simulink model "soc"  (R2025b)
settings: Solver=FixedStepDiscrete  StartTime=0.0  StopTime=10  FixedStep=0.01  RelTol=1e-3
PreLoadFcn:
  | % === Get the current model's directory ===
  | modelFullPath = get_param(bdroot, 'FileName');
  | modelDir = fileparts(modelFullPath);
  | 
  | 
  | % === Get the project root folder ===
  | projectRoot = fileparts(modelDir);
  | 
  | 
  | % === Add key folders to path ===
  | addpath(fullfile(projectRoot, 'ReferenceSubsystems'));
  | %addpath(fullfile(projectRoot, 'Docs'));
  | addpath(fullfile(projectRoot, 'design'));
  | 
  | 
  | % Load lookup table script
  | %run('Lookuptable.m');
  | 
  | 
  | 
  | 
PostLoadFcn:
  | float32 = Simulink.AliasType;
  | 
  | float32.BaseType = 'single';
  | 
  | float32.HeaderFile = 'Platform_Types.h';
  | 
  | assignin('base', 'float32', float32);
values from neighbouring files (symbols this model uses):
  Battsm_State_t : value not decoded    [soc.sldd]
  FRACTION_TO_PERCENT = 100.0    [soc.sldd]
  KeSoc_A_RestingCurrent = 4.0    [soc.sldd]
  KeSoc_frc_BotmOfDchRst = 0.0    [soc.sldd]
  KeSoc_frc_LowSocResetThd = 0.12    [soc.sldd]
  KeSoc_frc_LowSocSetThd = 0.1    [soc.sldd]
  KeSoc_frc_SocMaxLim = 1.0    [soc.sldd]
  KeSoc_frc_SocMinLim = 0.0    [soc.sldd]
  KeSoc_frc_TopOfChrgRst = 1.0    [soc.sldd]
  KeSoc_frc_UserSocMaxLim = 0.99    [soc.sldd]
  KeSoc_frc_UserSocMinLim = 0.014    [soc.sldd]
  KeSoc_nu_EpsVal = 2.2204460492503131E-16    [soc.sldd]
  KeSoc_nu_RestTauFactor = 3.0    [soc.sldd]
  KeSoc_sec_SampleTime = 0.01    [soc.sldd]
  KeSoc_sec_SocBodSetTime = 0.0    [soc.sldd]
  KeSoc_sec_SocTocSetTime = 0.0    [soc.sldd]
  KeSoc_V_BodMinCellVolt = 2.993    [soc.sldd]
  KeSoc_V_TocAvrgCellVolt = 4.5    [soc.sldd]
  KeSoc_V_TocMaxCellVolt = 4.5    [soc.sldd]
  PERCENT_TO_FRACTION = 0.01    [soc.sldd]
  SEC_TO_MILLISEC = 1000.0    [soc.sldd]
  SOC_NUM_OF_CELLS = 8.0    [soc.sldd]
  Soc_State_t : value not decoded    [soc.sldd]
libraries: simulink x25
(part 2 of 2)

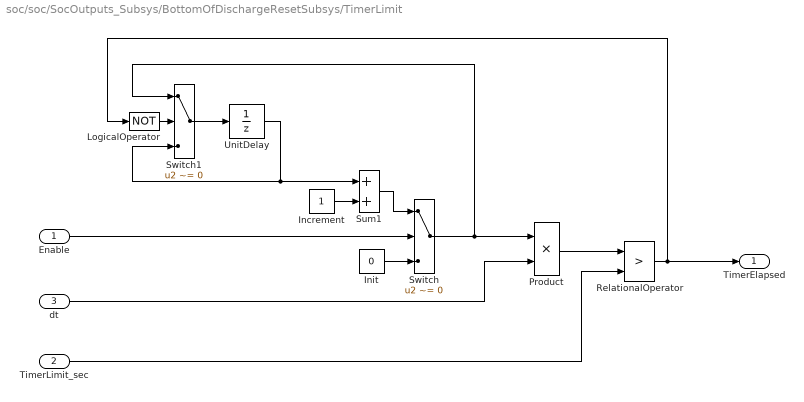
== system soc/soc/SocOutputs_Subsys/BottomOfDischargeResetSubsys/TimerLimit ==
  Enable : Inport  OutDataTypeStr=boolean
  TimerLimit_sec : Inport  Port=2
  dt : Inport  Port=3
  Increment : Constant  OutDataTypeStr=single  SampleTime=-1  FramePeriod=-1
  Init : Constant  Value=0  OutDataTypeStr=single  SampleTime=-1  FramePeriod=-1
  LogicalOperator : Logic  Operator=NOT  AllPortsSameDT=off  OutDataTypeStr=boolean
  Product : Product
  RelationalOperator : RelationalOperator  Tag=struct('comment',struct('text','','placement',1),'logdata',struct('maxnumvals',inf,'plotchannels',[],'stepsize',0,'downsampling',1,'loggingmode',3,'channels',1),'operator','>','output',struct('class','default','type','Bool','description','','address','','unit','','name','$S_$B'),'date',731828.013278403)  Operator=>  OutDataTypeStr=boolean
  Sum1 : Sum  Tag=struct('comment',struct('text','','placement',1),'logdata',struct('maxnumvals',inf,'plotchannels',[],'stepsize',0,'downsampling',1,'loggingmode',3,'channels',1),'output',struct('width',1,'name','$S_$B','unit','','type','Int16','offset',0,'max',NaN,'min',NaN,'freeze',1,'lsb',0.01,'arb',1,'class','default','address','','description','','autoscalingmode',1,'lowerheadroom',1,'upperheadroom',1,'headroomunit','bit','checkmin',0,'checkmax',1,'show',0),'inputs','++','date',731828.013278981)  InputSameDT=on  OutDataTypeStr=Inherit: Same as first input
  Switch : Switch  Tag=struct('comment',struct('text','','placement',1),'logdata',struct('maxnumvals',inf,'plotchannels',[],'stepsize',0,'downsampling',1,'loggingmode',3,'channels',1),'output',struct('width',1,'name','$S_$B','unit','','type','Int16','offset',0,'max',NaN,'min',NaN,'freeze',1,'lsb',0.01,'arb',1,'class','default','address','','description','','autoscalingmode',1,'lowerheadroom',1,'upperheadroom',1,'headroomunit','bit','checkmin',0,'checkmax',0,'show',0),'threshold',struct('width',1,'name','$S_$B_threshold','unit','','type','Int16','offset',0,'max',NaN,'min',NaN,'freeze',1,'lsb',1,'arb',0,'class','default','address','','description','','value','1','scalar',0),'date',731832.69671603)  Criteria=u2 ~= 0  OutDataTypeStr=Inherit: Inherit via back propagation  SaturateOnIntegerOverflow=off
      settings: AttributesFormatString=<Threshold = %<Threshold>>
  Switch1 : Switch  Tag=struct('comment',struct('text','','placement',1),'logdata',struct('maxnumvals',inf,'plotchannels',[],'stepsize',0,'downsampling',1,'loggingmode',3,'channels',1),'output',struct('width',1,'name','$S_$B','unit','','type','Int16','offset',0,'max',NaN,'min',NaN,'freeze',1,'lsb',0.01,'arb',1,'class','default','address','','description','','autoscalingmode',1,'lowerheadroom',1,'upperheadroom',1,'headroomunit','bit','checkmin',0,'checkmax',0,'show',0),'threshold',struct('width',1,'name','$S_$B_threshold','unit','','type','Int16','offset',0,'max',NaN,'min',NaN,'freeze',1,'lsb',1,'arb',0,'class','default','address','','description','','value','1','scalar',0),'date',731832.69671603)  Criteria=u2 ~= 0  OutDataTypeStr=Inherit: Inherit via back propagation  SaturateOnIntegerOverflow=off
      settings: AttributesFormatString=<Threshold = %<Threshold>>
  UnitDelay : UnitDelay  SampleTime=-1  HasFrameUpgradeWarning=on
      settings: AttributesFormatString=<IC: %<InitialCondition>>
  TimerElapsed : Outport  OutDataTypeStr=boolean  VectorParamsAs1DForOutWhenUnconnected=off
      settings: AttributesFormatString=|
      | <IC: %<InitialOutput>>
      | <%<OutputWhenDisabled>>
  wires:
  Increment/1 -> Sum1/2
  TimerLimit_sec/1 -> RelationalOperator/2
  RelationalOperator/1 -> LogicalOperator/1, TimerElapsed/1
  Switch1/1 -> UnitDelay/1
  dt/1 -> Product/2
  Init/1 -> Switch/3
  UnitDelay/1 -> Sum1/1, Switch1/3
  Sum1/1 -> Switch/1
  Product/1 -> RelationalOperator/1
  LogicalOperator/1 -> Switch1/2
  Switch/1 -> Product/1, Switch1/1
  Enable/1 -> Switch/2

== system soc/soc/SocOutputs_Subsys/CalculatePackSoc_Subsys/CapacityRemaining ==
  VaSoc_pct_CellSoc : Inport
  VaSoc_frc_CellSohc : Inport  Port=2
  Constant : Constant  Value=KeSoc_frc_SocMinLim
  Min1 : MinMax  OutMin=0.01  OutMax=1
  Product : Product
  Subtract : Sum  Inputs=+-
  LeSoc_nu_CapcRemaining : Outport  OutMin=0.01  OutMax=1
  wires:
  VaSoc_pct_CellSoc/1 -> Subtract/1
  Constant/1 -> Subtract/2
  Subtract/1 -> Product/1
  VaSoc_frc_CellSohc/1 -> Product/2
  Product/1 -> Min1/1
  Min1/1 -> LeSoc_nu_CapcRemaining/1  "LeSoc_nu_CapcRemaining"

== system soc/soc/SocOutputs_Subsys/CalculatePackSoc_Subsys/CapacityToFullCharge ==
  VaSoc_pct_CellSoc : Inport
  VaSoc_frc_CellSohc : Inport  Port=2
  KeSoc_frc_SocMaxLim : Constant  Value=KeSoc_frc_SocMaxLim
  Min : MinMax  OutMin=0.01  OutMax=1
  Product : Product
  Subtract : Sum  Inputs=+-
  LeSoc_frc_CapcToFullChrg : Outport  OutMin=0.01  OutMax=1
  wires:
  KeSoc_frc_SocMaxLim/1 -> Subtract/1
  VaSoc_pct_CellSoc/1 -> Subtract/2
  Subtract/1 -> Product/1
  VaSoc_frc_CellSohc/1 -> Product/2
  Product/1 -> Min/1
  Min/1 -> LeSoc_frc_CapcToFullChrg/1  "LeSoc_frc_CapcToFullChrg"

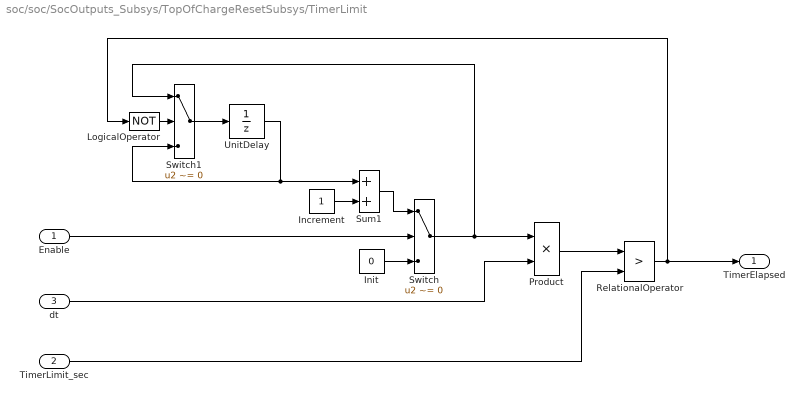
== system soc/soc/SocOutputs_Subsys/TopOfChargeResetSubsys/TimerLimit ==
  Enable : Inport  OutDataTypeStr=boolean
  TimerLimit_sec : Inport  Port=2
  dt : Inport  Port=3
  Increment : Constant  OutDataTypeStr=single  SampleTime=-1  FramePeriod=-1
  Init : Constant  Value=0  OutDataTypeStr=single  SampleTime=-1  FramePeriod=-1
  LogicalOperator : Logic  Operator=NOT  AllPortsSameDT=off  OutDataTypeStr=boolean
  Product : Product
  RelationalOperator : RelationalOperator  Tag=struct('comment',struct('text','','placement',1),'logdata',struct('maxnumvals',inf,'plotchannels',[],'stepsize',0,'downsampling',1,'loggingmode',3,'channels',1),'operator','>','output',struct('class','default','type','Bool','description','','address','','unit','','name','$S_$B'),'date',731828.013278403)  Operator=>  OutDataTypeStr=boolean
  Sum1 : Sum  Tag=struct('comment',struct('text','','placement',1),'logdata',struct('maxnumvals',inf,'plotchannels',[],'stepsize',0,'downsampling',1,'loggingmode',3,'channels',1),'output',struct('width',1,'name','$S_$B','unit','','type','Int16','offset',0,'max',NaN,'min',NaN,'freeze',1,'lsb',0.01,'arb',1,'class','default','address','','description','','autoscalingmode',1,'lowerheadroom',1,'upperheadroom',1,'headroomunit','bit','checkmin',0,'checkmax',1,'show',0),'inputs','++','date',731828.013278981)  InputSameDT=on  OutDataTypeStr=Inherit: Same as first input
  Switch : Switch  Tag=struct('comment',struct('text','','placement',1),'logdata',struct('maxnumvals',inf,'plotchannels',[],'stepsize',0,'downsampling',1,'loggingmode',3,'channels',1),'output',struct('width',1,'name','$S_$B','unit','','type','Int16','offset',0,'max',NaN,'min',NaN,'freeze',1,'lsb',0.01,'arb',1,'class','default','address','','description','','autoscalingmode',1,'lowerheadroom',1,'upperheadroom',1,'headroomunit','bit','checkmin',0,'checkmax',0,'show',0),'threshold',struct('width',1,'name','$S_$B_threshold','unit','','type','Int16','offset',0,'max',NaN,'min',NaN,'freeze',1,'lsb',1,'arb',0,'class','default','address','','description','','value','1','scalar',0),'date',731832.69671603)  Criteria=u2 ~= 0  OutDataTypeStr=Inherit: Inherit via back propagation  SaturateOnIntegerOverflow=off
      settings: AttributesFormatString=<Threshold = %<Threshold>>
  Switch1 : Switch  Tag=struct('comment',struct('text','','placement',1),'logdata',struct('maxnumvals',inf,'plotchannels',[],'stepsize',0,'downsampling',1,'loggingmode',3,'channels',1),'output',struct('width',1,'name','$S_$B','unit','','type','Int16','offset',0,'max',NaN,'min',NaN,'freeze',1,'lsb',0.01,'arb',1,'class','default','address','','description','','autoscalingmode',1,'lowerheadroom',1,'upperheadroom',1,'headroomunit','bit','checkmin',0,'checkmax',0,'show',0),'threshold',struct('width',1,'name','$S_$B_threshold','unit','','type','Int16','offset',0,'max',NaN,'min',NaN,'freeze',1,'lsb',1,'arb',0,'class','default','address','','description','','value','1','scalar',0),'date',731832.69671603)  Criteria=u2 ~= 0  OutDataTypeStr=Inherit: Inherit via back propagation  SaturateOnIntegerOverflow=off
      settings: AttributesFormatString=<Threshold = %<Threshold>>
  UnitDelay : UnitDelay  SampleTime=-1  HasFrameUpgradeWarning=on
      settings: AttributesFormatString=<IC: %<InitialCondition>>
  TimerElapsed : Outport  OutDataTypeStr=boolean  VectorParamsAs1DForOutWhenUnconnected=off
      settings: AttributesFormatString=|
      | <IC: %<InitialOutput>>
      | <%<OutputWhenDisabled>>
  wires:
  Increment/1 -> Sum1/2
  TimerLimit_sec/1 -> RelationalOperator/2
  RelationalOperator/1 -> LogicalOperator/1, TimerElapsed/1
  Switch1/1 -> UnitDelay/1
  dt/1 -> Product/2
  Init/1 -> Switch/3
  UnitDelay/1 -> Sum1/1, Switch1/3
  Sum1/1 -> Switch/1
  Product/1 -> RelationalOperator/1
  LogicalOperator/1 -> Switch1/2
  Switch/1 -> Product/1, Switch1/1
  Enable/1 -> Switch/2

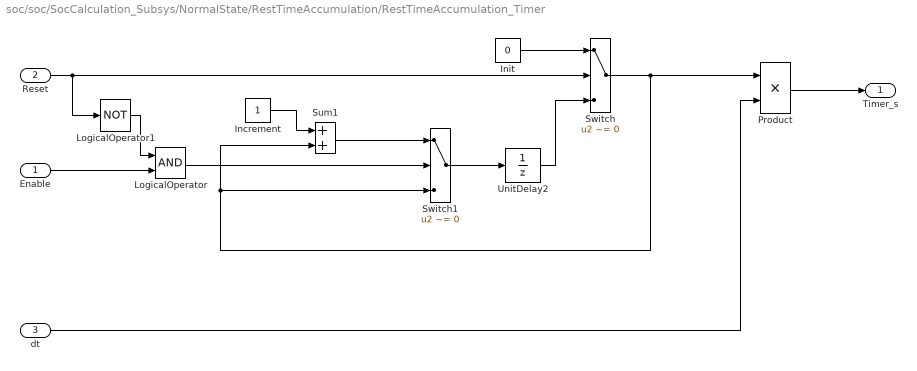
== system soc/soc/SocCalculation_Subsys/NormalState/RestTimeAccumulation/RestTimeAccumulation_Timer ==
  Enable : Inport
  Reset : Inport  Port=2
  dt : Inport  Port=3
  Increment : Constant  OutDataTypeStr=single  SampleTime=-1  FramePeriod=-1
  Init : Constant  Value=0  OutDataTypeStr=single  SampleTime=-1  FramePeriod=-1
  LogicalOperator : Logic  AllPortsSameDT=off  OutDataTypeStr=boolean
  LogicalOperator1 : Logic  Operator=NOT  AllPortsSameDT=off  OutDataTypeStr=boolean
  Product : Product
  Sum1 : Sum  Tag=struct('comment',struct('text','','placement',1),'logdata',struct('maxnumvals',inf,'plotchannels',[],'stepsize',0,'downsampling',1,'loggingmode',3,'channels',1),'output',struct('width',1,'name','$S_$B','unit','','type','Int16','offset',0,'max',NaN,'min',NaN,'freeze',1,'lsb',0.01,'arb',1,'class','default','address','','description','','autoscalingmode',1,'lowerheadroom',1,'upperheadroom',1,'headroomunit','bit','checkmin',0,'checkmax',1,'show',0),'inputs','++','date',731828.013278981)  InputSameDT=on  OutDataTypeStr=Inherit: Same as first input
  Switch : Switch  Criteria=u2 ~= 0  OutDataTypeStr=Inherit: Inherit via back propagation  SaturateOnIntegerOverflow=off
      settings: AttributesFormatString=<Threshold = %<Threshold>>
  Switch1 : Switch  Criteria=u2 ~= 0  OutDataTypeStr=Inherit: Inherit via back propagation  SaturateOnIntegerOverflow=off
      settings: AttributesFormatString=<Threshold = %<Threshold>>
  UnitDelay2 : UnitDelay  SampleTime=-1  HasFrameUpgradeWarning=on
      settings: AttributesFormatString=<IC: %<InitialCondition>>
  Timer_s : Outport  OutDataTypeStr=single  InitialOutput=[0]  VectorParamsAs1DForOutWhenUnconnected=off
      settings: AttributesFormatString=|
      | <IC: %<InitialOutput>>
      | <%<OutputWhenDisabled>>
  wires:
  Enable/1 -> LogicalOperator/2
  Reset/1 -> Switch/2, LogicalOperator1/1
  dt/1 -> Product/2
  Increment/1 -> Sum1/1
  Switch/1 -> Product/1, Sum1/2, Switch1/3
  Switch1/1 -> UnitDelay2/1
  LogicalOperator1/1 -> LogicalOperator/1
  Sum1/1 -> Switch1/1
  Product/1 -> Timer_s/1
  LogicalOperator/1 -> Switch1/2
  Init/1 -> Switch/1
  UnitDelay2/1 -> Switch/3

== stateflow chart soc/SocStateMachine_Subsys/SOC_StateMachine_Chart ==
  note: SOC State Machine:
  state INIT_STATE
    en:
    LeSoc_nu_SocSt=Soc_State_t.SOC_STATE_INIT;
    LeSoc_bi_SocInNormalStateFlg=false;
  note: SOC state machine description:
      |
      | SOC States: SOC_STATE_INIT -0 (Default state)
      | SOC_STATE_RESET - 1
      | SOC_STATE_CORRECTION_ON_WAKE - 2
      | SOC_STATE_NORMAL - 3
      |
      | INIT STATE:
      | This is the default state where the algorithm initializes the SOC values using the data imported from NVM.
      | Based on the NeSoc_bi_NvmImprtScsf flag and the current battery state, the state machine transitions to either SOC_Correction_on_Wake or SOC_Reset.
      |
      | SOC RESET STATE:
      | If the NVM import fails, the SOC values are reset or reinitialized using OCV-based estimates, and the rest time is set to zero.
      | The system then transitions to the Normal state once the battery enters Charge or Drive mode.
      |
      | SOC CORRECTION ON WAKE STATE:
      | If the NVM import is successful, the algorithm checks for any previously accumulated rest time that may require SOC correction before entering the Normal state.
      | If the rest time is sufficiently long, SOC correction is performed; otherwise, the SOC value imported from NVM is retained as the initial SOC.
      | The state transitions to Normal when the battery is in Charge or Drive mode.
      |
      | NORMAL STATE:
      | In this state, SOC is computed using the coulomb counting method.
      | If the battery enters a rest condition, the rest time is accumulated.
      | Once the accumulated rest time exceeds the defined threshold, SOC correction is performed, and the updated value is stored
  state CORRECTION_ON_WAKE_STATE
    en:
    LeSoc_nu_SocSt=Soc_State_t.SOC_STATE_CORRECTION_ON_WAKE;
  state RESET_STATE
    en:
    LeSoc_nu_SocSt=Soc_State_t.SOC_STATE_RESET;
  state NORMAL_STATE
    en:
    LeSoc_nu_SocSt=Soc_State_t.SOC_STATE_NORMAL;
    du:
    LeSoc_bi_SocInNormalStateFlg=true;
    if LeSoc_bi_RestCorrCmpFlg
    LeSoc_bi_CcRst = true;
    else
    LeSoc_bi_CcRst = false;
    end
  (default) -> INIT_STATE
  INIT_STATE -> (junction 8) [order 1] : [NeSoc_bi_NvmImprtScsf == true &&...
      | [ VeBattsm_nu_BattState == Battsm_State_t.BATTSM_STATE_STANDBY_INIT ||...
      | VeBattsm_nu_BattState == Battsm_State_t.BATTSM_STATE_STANDBY_NOT_READY ||...
      | VeBattsm_nu_BattState == Battsm_State_t.BATTSM_STATE_STANDBY_READY]]
  (junction 8) -> CORRECTION_ON_WAKE_STATE
  INIT_STATE -> RESET_STATE [order 2] : [NeSoc_bi_NvmImprtScsf ~= true &&...
      | [ VeBattsm_nu_BattState == Battsm_State_t.BATTSM_STATE_STANDBY_INIT ||...
      | VeBattsm_nu_BattState == Battsm_State_t.BATTSM_STATE_STANDBY_NOT_READY ||...
      | VeBattsm_nu_BattState == Battsm_State_t.BATTSM_STATE_STANDBY_READY]]
  RESET_STATE -> (junction 42) : [LeSoc_bi_SocRstCmplFlg == true &&...
      | [VeBattsm_nu_BattState == Battsm_State_t.BATTSM_STATE_CHARGE ||...
      |  VeBattsm_nu_BattState == Battsm_State_t.BATTSM_STATE_DRIVE]]
  CORRECTION_ON_WAKE_STATE -> (junction 44) : [LeSoc_bi_SocCorrnOnWkCmplFlg == true &&...
      | [VeBattsm_nu_BattState == Battsm_State_t.BATTSM_STATE_CHARGE ||...
      |  VeBattsm_nu_BattState == Battsm_State_t.BATTSM_STATE_DRIVE]]
  (junction 42) -> NORMAL_STATE
  (junction 44) -> NORMAL_STATE
  data: NeSoc_bi_NvmImprtScsf input boolean; LeSoc_nu_SocSt output Enum: Soc_State_t =Soc_State_t.SOC_STATE_INIT; LeSoc_bi_SocCorrnOnWkCmplFlg input boolean; LeSoc_bi_SocRstCmplFlg input boolean; VeBattsm_nu_BattState input Enum: Battsm_State_t; LeSoc_bi_CcRst output boolean; LeSoc_bi_RestCorrCmpFlg input boolean; LeSoc_bi_SocInNormalStateFlg output boolean
  data LeSoc_bi_CcRst settings: description=Reset pulse for CC integrator
